simulink library "tp333079"  (Simulink 5.0)
values from neighbouring files (symbols this model uses):
  b = 1    [main_flock3.m]    (also in main_flock4.m; params_flocking_ros.m)
undefined symbols (not defined in the file or in its folder): AC, AlphaBnd, BetaBnd, CDda, CDde, CDdf, CDdr, CDM, CDmin, CGempty, CGgross, CL0, CLa, CLalphadot, Clbeta, Clda, CLde, CLdf, Cldr, CLM, CLmind, Clp, CLq, Clr, Cm0, Cma, Cmalphadot, Cmde, Cmdf, CmM, Cmq, Cnbeta, Cnda, Cndr, Cnp, Cnr, CP, CT, CYbeta, CYda, CYdr, CYp, CYr, Displacement, dmy, Engine, EulerIni, FuelFlow, FuelIni, J, Jempty, Jeng, Jgross, Jprop, MAC, MAP, MAPLim, MassIni, MaxPower, mempty ... (+26)
libraries: aerosimlib x325, simulink3 x42
(part 4 of 11)

== system tp333079/FlightGear-Compatible/Complete Aircraft ==
  CESSNA-172 : Subsystem  SimViewingDevice=off  mask(FlightGear Aircraft Model){ACName='c172', FGPath='f:\flightgear-0.8', VelocitiesIni=[60 0 0]', RatesIni=[0 0 0]', QuaternionsIni=[1 0 0 0]', PositionIni=[37.6*pi/180 -122.3*pi/180 2000]', OmegaIni=2500*pi/30, FuelIni=[50 50], GndAlt=0, tsamp=0.02}
      mask prompts: ACName "Aircraft name:"; FGPath "FlightGear path:"; VelocitiesIni "Initial velocities:"; RatesIni "Initial angular rate:"; QuaternionsIni "Initial quaternions:"; PositionIni "Initial position:"; OmegaIni "Initial engine speed:"; FuelIni "Initial fuel:"; GndAlt "Ground altitude:"; tsamp "Sample time:"
      mask help: A FlightGear aircraft model, with single piston engine, fixed-pitch propeller, and two fuel tanks.
      mask init:
      | ACen = xmlAircraft(ACName, FGPath);
      | AC = AircraftUnitConv(ACen);
      settings: Permissions=ReadWrite  RTWFcnNameOpts=Auto  RTWFileNameOpts=Auto
      mask Help:
      | A FlightGear aircraft model, with single piston engine, fixed-pitch propeller, and two fuel tanks. All parameters are in metric units. Angular measurements are in radians.
      | <P><B>Inputs:</B>
      | <LI>Control = the aircraft control vector [Flap Elevator Aileron Rudder Throttle Mixture Ignition]</LI>
      | <LI>Wind = the background wind vector, in geodetic frame [WN WE WD]</LI>
      | <LI>RST = the integrator reset flag</LI>
      | </P>
      | <P><B>Outputs:</B>
      | <LI>TAS = the true airspeed</LI>
      | <LI>AOA = the angle-of-attack</LI>
      | <LI>Position = the aircraft position [Lat Lon Alt]</LI>
      | <LI>Attitude = the aircraft attitude in Euler angles [roll pitch yaw]</LI>
      | <LI>Rates = the angular rates in body axes</LI>
      | <LI>Aero = the aerodynamic coefficients [CD CY CL Cl Cm Cn]</LI>
      | <LI>Prop = the propeller coefficients [J CT CP]</LI>
      | <LI>Engine = the engine coefficients [MAP AF FF BSFC P]</LI>
      | <LI>RPM = the engine rotation speed</LI>
      | </P>
      | <P><B>Parameters:</B>
      | <LI>Aircraft name = the name of the JSBSim aircraft</LI>
      | <LI>FlightGear path</LI>
      | <LI>Initial velocities</LI>
      | <LI>Initial angular rates</LI>
      | <LI>Initial quaternions</LI>
      | <LI>Initial position</LI>
      | <LI>Initial engine speed</LI>
      | <LI>Initial fuel mass</LI>
      | <LI>Ground altitude</LI>
      | <LI>Sample time</LI>
      | </P>
  CESSNA-182 : Subsystem  SimViewingDevice=off  mask(FlightGear Aircraft Model){ACName='c182', FGPath='f:\flightgear-0.8', VelocitiesIni=[70 0 0]', RatesIni=[0 0 0]', QuaternionsIni=[1 0 0 0]', PositionIni=[37.6*pi/180 -122.3*pi/180 500]', OmegaIni=2500*pi/30, FuelIni=[100 100], GndAlt=0, tsamp=0.02}
      mask prompts: ACName "Aircraft name:"; FGPath "FlightGear path:"; VelocitiesIni "Initial velocities:"; RatesIni "Initial angular rate:"; QuaternionsIni "Initial quaternions:"; PositionIni "Initial position:"; OmegaIni "Initial engine speed:"; FuelIni "Initial fuel:"; GndAlt "Ground altitude:"; tsamp "Sample time:"
      mask help: A FlightGear aircraft model, with single piston engine, variable-pitch propeller, and two fuel tanks.
      mask init:
      | ACen = xmlAircraft(ACName, FGPath);
      | AC = AircraftUnitConv(ACen);
      settings: Permissions=ReadWrite  RTWFcnNameOpts=Auto  RTWFileNameOpts=Auto
      mask Help:
      | A FlightGear aircraft model, with single piston engine, variable-pitch propeller, and two fuel tanks.
      | <P><B>Inputs:</B>
      | <LI>Control = the aircraft control vector [Flap Elevator Aileron Rudder Throttle Mixture Ignition Prop-pitch]</LI>
      | <LI>Wind = the background wind vector, in geodetic frame [WN WE WD]</LI>
      | <LI>RST = the integrator reset flag</LI>
      | </P>
      | <P><B>Outputs:</B>
      | <LI>TAS = the true airspeed</LI>
      | <LI>AOA = the angle-of-attack</LI>
      | <LI>Position = the aircraft position [Lat Lon Alt]</LI>
      | <LI>Attitude = the aircraft attitude in Euler angles [roll pitch yaw]</LI>
      | <LI>Rates = the angular rates in body axes</LI>
      | <LI>Aero = the aerodynamic coefficients [CD CY CL Cl Cm Cn]</LI>
      | <LI>Prop = the propeller coefficients [J CT CP]</LI>
      | <LI>Engine = the engine coefficients [MAP AF FF BSFC P]</LI>
      | <LI>RPM = the engine rotation speed</LI>
      | </P>
      | <P><B>Parameters:</B>
      | <LI>Aircraft name = the name of the JSBSim aircraft</LI>
      | <LI>FlightGear path</LI>
      | <LI>Initial velocities</LI>
      | <LI>Initial angular rates</LI>
      | <LI>Initial quaternions</LI>
      | <LI>Initial position</LI>
      | <LI>Initial engine speed</LI>
      | <LI>Initial fuel mass</LI>
      | <LI>Ground altitude</LI>
      | <LI>Sample time</LI>
      | </P>
  CESSNA-310 : Subsystem  SimViewingDevice=off  mask(FlightGear Aircraft Model){ACName='c310', FGPath='f:\flightgear-0.8', VelocitiesIni=[90 0 0]', RatesIni=[0 0 0]', QuaternionsIni=[1 0 0 0]', PositionIni=[37.6*pi/180 -122.3*pi/180 500]', OmegaIni=[2500 2500]*pi/30, FuelIni=[100 100 50 50], GndAlt=0, tsamp=0.02}
      mask prompts: ACName "Aircraft name:"; FGPath "FlightGear path:"; VelocitiesIni "Initial velocities:"; RatesIni "Initial angular rate:"; QuaternionsIni "Initial quaternions:"; PositionIni "Initial position:"; OmegaIni "Initial engine speed:"; FuelIni "Initial fuel:"; GndAlt "Ground altitude:"; tsamp "Sample time:"
      mask help: A FlightGear aircraft model, twin engine, variable-pitch propellers, and 4 fuel tanks.
      mask init:
      | ACen = xmlAircraft(ACName, FGPath);
      | AC = AircraftUnitConv(ACen);
      settings: Permissions=ReadWrite  RTWFcnNameOpts=Auto  RTWFileNameOpts=Auto
      mask Help:
      | A FlightGear aircraft model, twin engine, variable-pitch propellers, and 4 fuel tanks.
      | <P><B>Inputs:</B>
      | <LI>Control = the aircraft control vector [Flap Elevator Aileron Rudder ThrottleL MixtureL IgnitionL Prop-pitchL ThrottleR MixtureR IgnitionR Prop-pitchR]</LI>
      | <LI>Gear = the gear position flag (0 = gear up, 1 = gear down)</LI>
      | <LI>Wind = the background wind vector, in geodetic frame [WN WE WD]</LI>
      | <LI>RST = the integrator reset flag</LI>
      | </P>
      | <P><B>Outputs:</B>
      | <LI>TAS = the true airspeed</LI>
      | <LI>AOA = the angle-of-attack</LI>
      | <LI>Position = the aircraft position [Lat Lon Alt]</LI>
      | <LI>Attitude = the aircraft attitude in Euler angles [roll pitch yaw]</LI>
      | <LI>Rates = the angular rates in body axes</LI>
      | <LI>Aero = the aerodynamic coefficients [CD CY CL Cl Cm Cn]</LI>
      | <LI>PropL = the left propeller coefficients [J CT CP]</LI>
      | <LI>EngineL = the left engine coefficients [MAP AF FF BSFC P]</LI>
      | <LI>RPML = the left engine rotation speed</LI>
      | <LI>PropR = the right propeller coefficients [J CT CP]</LI>
      | <LI>EngineR = the right engine coefficients [MAP AF FF BSFC P]</LI>
      | <LI>RPMR = the right engine rotation speed</LI>
      | </P>
      | <P><B>Parameters:</B>
      | <LI>Aircraft name = the name of the JSBSim aircraft</LI>
      | <LI>FlightGear path</LI>
      | <LI>Initial velocities</LI>
      | <LI>Initial angular rates</LI>
      | <LI>Initial quaternions</LI>
      | <LI>Initial position</LI>
      | <LI>Initial engine speed [left eng, right eng]</LI>
      | <LI>Initial fuel mass [inner left, inner right, outer left, outer right]</LI>
      | <LI>Ground altitude</LI>
      | <LI>Sample time</LI>
      | </P>

== system tp333079/FlightGear-Compatible/Inertia ==
  Empty Aircraft : Subsystem  SimViewingDevice=off  mask(Empty Aircraft){Metrics=Metrics}
      mask prompts: Metrics "Aircraft metrics structure:"
      mask help: The block returns the empty aircraft inertia parameters (mass, CG location, and moments of inertia Jx Jy Jz and Jxz).
      settings: Permissions=ReadWrite  RTWFcnNameOpts=Auto  RTWFileNameOpts=Auto
      mask Help:
      | The block returns the empty aircraft inertia parameters (mass, CG location, and moments of inertia Jx Jy Jz and Jxz).
      | <P><B>Inputs:</B>
      | <LI>none</LI>
      | </P>
      | <P><B>Outputs:</B>
      | <LI>Mass = the empty aircraft mass</LI>
      | <LI>CG = the empty aircraft CG location [x y z]</LI>
      | <LI>Inertia = the empty aircraft moments of inertia [Jx Jy Jz Jxz]</LI>
      | </P>
      | <P><B>Parameters:</B>
      | <LI>Aircraft metrics structure = the Matlab structure which describes the aircraft metrics (part of the aircraft structure)</LI>
      | </P>
  Point Mass : Subsystem  SimViewingDevice=off  mask(Point Mass){PointMass=PointMass}
      mask prompts: PointMass "Point mass structure:"
      mask help: The block returns the inertia parameters of a point-mass component.
      settings: Permissions=ReadWrite  RTWFcnNameOpts=Auto  RTWFileNameOpts=Auto
      mask Help:
      | The block returns the inertia parameters of a point-mass component (mass, CG location, and moments of inertia Jx Jy Jz and Jxz).
      | <P><B>Inputs:</B>
      | <LI>none</LI>
      | </P>
      | <P><B>Outputs:</B>
      | <LI>Mass = the component mass</LI>
      | <LI>CG = the component CG location [x y z]</LI>
      | <LI>Inertia = the component moments of inertia [Jx Jy Jz Jxz]</LI>
      | </P>
      | <P><B>Parameters:</B>
      | <LI>Point mass structure = the Matlab structure which describes the point mass component (part of the aircraft structure)</LI>
      | </P>

== system tp333079/FlightGear-Compatible/Propulsion ==
  Engine : Subsystem  SimViewingDevice=off
      settings: Permissions=ReadWrite  RTWFcnNameOpts=Auto  RTWFileNameOpts=Auto
  FG Piston Engine +  Fixed-Pitch Prop : Subsystem  SimViewingDevice=off  mask(FG Piston Engine + Fixed-Pitch Prop){Eng=Engine, Thr=Thruster, pSL=pSL, TSL=TSL, OmegaIni=OmegaIni}
      mask prompts: Eng "Piston engine structure:"; Thr "Fixed-pitch prop structure:"; pSL "Sea-level pressure:"; TSL "Sea-level temperature:"; OmegaIni "Initial engine speed:"
      mask help: The block includes a piston engine, a fixed-pitch propeller and the propulsion system moment equation.
      settings: Permissions=ReadWrite  RTWFcnNameOpts=Auto  RTWFileNameOpts=Auto
      mask Help:
      | The block includes a piston engine, a fixed-pitch propeller and the propulsion system moment equation.
      | <P><B>Inputs:</B>
      | <LI>Control = the engine controls [Throttle Mixture Ignition]</LI>
      | <LI>p = the atmospheric pressure</LI>
      | <LI>T = the outside air temperature</LI>
      | <LI>rho = the air density at current altitude</LI>
      | <LI>WindAxesVel = the aircraft velocity in wind axes [airspeed sideslip angle-of-attack]</LI>
      | <LI>CGpos = the current location of the aircraft center of gravity</LI>
      | <LI>RST = the engine speed integrator reset flag</LI>
      | </P>
      | <P><B>Outputs:</B>
      | <LI>Fprop = the propulsion forces in body axes</LI>
      | <LI>Mprop = the propulsion moments with respect to the current aircraft CG</LI>
      | <LI>Omega = the engine rotation speed</LI>
      | <LI>FuelFlow = the mass fuel flow to the engine</LI>
      | <LI>EngCoeff = the engine coefficients [MAP AirFlow FuelFlow BSFC Power]</LI>
      | <LI>PropCoeff = the propeller coefficients [J CT CP]</LI>
      | </P>
      | <P><B>Parameters:</B>
      | <LI>Piston engine structure = the Matlab engine structure, which is part of the aircraft structure</LI>
      | <LI>Fixed-pitch prop structure = the Matlab thruster structure, which is part of the aircraft structure</LI>
      | <LI> Sea-level pressure and temperature</LI>
      | <LI>Initial engine speed = the initial value for the engine speed integrator</LI>
      | </P>
  FG Piston Engine +  Variable-Pitch Prop : Subsystem  SimViewingDevice=off  mask(FG Piston Engine + Variable-Pitch Prop){Eng=AC.Propulsion.Engine{1}, Thr=AC.Propulsion.Thruster{1}, pSL=101325, TSL=288.15, OmegaIni=OmegaIni}
      mask prompts: Eng "Piston engine structure:"; Thr "Fixed-pitch prop structure:"; pSL "Sea-level pressure:"; TSL "Sea-level temperature:"; OmegaIni "Initial engine speed:"
      mask help: The block includes a piston engine, a variable-pitch propeller and the propulsion system moment equation.
      settings: Permissions=ReadWrite  RTWFcnNameOpts=Auto  RTWFileNameOpts=Auto
      mask Help:
      | The block includes a piston engine, a variable-pitch propeller and the propulsion system moment equation.
      | <P><B>Inputs:</B>
      | <LI>Control = the engine controls [Throttle Mixture Ignition Prop-pitch]</LI>
      | <LI>p = the atmospheric pressure</LI>
      | <LI>T = the outside air temperature</LI>
      | <LI>rho = the air density at current altitude</LI>
      | <LI>WindAxesVel = the aircraft velocity in wind axes [airspeed sideslip angle-of-attack]</LI>
      | <LI>CGpos = the current location of the aircraft center of gravity</LI>
      | <LI>RST = the engine speed integrator reset flag</LI>
      | </P>
      | <P><B>Outputs:</B>
      | <LI>Fprop = the propulsion forces in body axes</LI>
      | <LI>Mprop = the propulsion moments with respect to the current aircraft CG</LI>
      | <LI>Omega = the engine rotation speed</LI>
      | <LI>FuelFlow = the mass fuel flow to the engine</LI>
      | <LI>EngCoeff = the engine coefficients [MAP AirFlow FuelFlow BSFC Power]</LI>
      | <LI>PropCoeff = the propeller coefficients [J CT CP]</LI>
      | </P>
      | <P><B>Parameters:</B>
      | <LI>Piston engine structure = the Matlab engine structure, which is part of the aircraft structure</LI>
      | <LI>Fixed-pitch prop structure = the Matlab thruster structure, which is part of the aircraft structure</LI>
      | <LI> Sea-level pressure and temperature</LI>
      | <LI>Initial engine speed = the initial value for the engine speed integrator</LI>
      | </P>
  Tank : Subsystem  SimViewingDevice=off
      settings: Permissions=ReadWrite  RTWFcnNameOpts=Auto  RTWFileNameOpts=Auto
  Thruster : Subsystem  SimViewingDevice=off
      settings: Permissions=ReadWrite  RTWFcnNameOpts=Auto  RTWFileNameOpts=Auto

== system tp333079/Inertia/Aircraft Inertia ==
  note: Interpolate to get current moments of inertia
  note: Interpolate to get current CG location
  note: Compute current aircraft mass
  FuelFlow : Inport  Port=1  PortDimensions=1  SampleTime=-1  DataType=auto
      settings: SignalType=auto
  RST : Inport  Port=2  PortDimensions=1  SampleTime=-1  DataType=auto
      settings: SignalType=auto
  CG Position X : Lookup  InputValues=[Mempty Mgross]  OutputValues=[CGempty(1) CGgross(1)]
  CG Position Y : Lookup  InputValues=[Mempty Mgross]  OutputValues=[CGempty(2) CGgross(2)]
  CG Position Z : Lookup  InputValues=[Mempty Mgross]  OutputValues=[CGempty(3) CGgross(3)]
  ChSign : Gain  Gain=-1  Multiplication=Element-wise(K.*u)  SaturateOnIntegerOverflow=on
  Fuel Integrator : Integrator  ExternalReset=rising  InitialConditionSource=internal  InitialCondition=FuelIni  LimitOutput=on  UpperSaturationLimit=Mgross-Mempty  LowerSaturationLimit=0  ShowSaturationPort=off  ShowStatePort=off  AbsoluteTolerance=auto
  Inertia Moment Jx : Lookup  InputValues=[Mempty Mgross]  OutputValues=[Jempty(1) Jgross(1)]
  Inertia Moment Jxz : Lookup  InputValues=[Mempty Mgross]  OutputValues=[Jempty(4) Jgross(4)]
  Inertia Moment Jy : Lookup  InputValues=[Mempty Mgross]  OutputValues=[Jempty(2) Jgross(2)]
  Inertia Moment Jz : Lookup  InputValues=[Mempty Mgross]  OutputValues=[Jempty(3) Jgross(3)]
  Mass empty : Constant  Value=Mempty
  Mux : Mux  Inputs=3
  Mux1 : Mux  Inputs=4
  Relational Operator : RelationalOperator  Operator===
  Sum : Sum  Inputs=|++  SaturateOnIntegerOverflow=on
  Fuel : Outport  Port=1
  Mass : Outport  Port=2
  CGpos : Outport  Port=3
  Inertia : Outport  Port=4
  OutofFuel : Outport  Port=5
  wires:
  Mux1/1 -> Inertia/1
  Inertia Moment Jxz/1 -> Mux1/4
  Inertia Moment Jz/1 -> Mux1/3
  Inertia Moment Jy/1 -> Mux1/2
  Inertia Moment Jx/1 -> Mux1/1
  CG Position Z/1 -> Mux/3
  CG Position Y/1 -> Mux/2
  CG Position X/1 -> Mux/1
  Sum/1 -> Mass/1, Inertia Moment Jy/1, Inertia Moment Jz/1, Inertia Moment Jxz/1, Inertia Moment Jx/1, CG Position Y/1, CG Position Z/1, CG Position X/1, Relational Operator/1
  Mass empty/1 -> Sum/2, Relational Operator/2
  Fuel Integrator/1 -> Sum/1, Fuel/1
  RST/1 -> Fuel Integrator/2
  ChSign/1 -> Fuel Integrator/1
  FuelFlow/1 -> ChSign/1
  Mux/1 -> CGpos/1
  Relational Operator/1 -> OutofFuel/1

== system tp333079/Inertia/Inertia Coefficients ==
  note: Output
  note: Get Gamma
  note: Sources
  Inertia : Inport  Port=1  PortDimensions=[4 1]  SampleTime=-1  DataType=auto
      settings: SignalType=auto
  (Jx-Jy+Jz)Jxz : Product  Inputs=2  Multiplication=Element-wise(.*)  SaturateOnIntegerOverflow=on
  (Jy-Jz)Jz : Product  Inputs=2  Multiplication=Element-wise(.*)  SaturateOnIntegerOverflow=on
  Demux : Demux  Outputs=4  BusSelectionMode=off
  Divide{,1..8} (9 alike) : Product  Inputs=*/  Multiplication=Element-wise(.*)  SaturateOnIntegerOverflow=on
  Jx(Jx-Jy) : Product  Inputs=2  Multiplication=Element-wise(.*)  SaturateOnIntegerOverflow=on
  JxJz : Product  Inputs=2  Multiplication=Element-wise(.*)  SaturateOnIntegerOverflow=on
  Jxz^2 : Math  Operator=square  OutputSignalType=auto
  Mux : Mux  Inputs=9
  One : Constant  Value=1
  Sum{,1..2,4..5} (5 alike) : Sum  Inputs=|+-  SaturateOnIntegerOverflow=on
  Sum3 : Sum  Inputs=+-+  SaturateOnIntegerOverflow=on
  Sum6 : Sum  Inputs=|++  SaturateOnIntegerOverflow=on
  Coeff : Outport  Port=1
  wires:
  Mux/1 -> Coeff/1
  Divide8/1 -> Mux/9
  Sum5/1 -> Jx(Jx-Jy)/2
  Divide7/1 -> Mux/8
  Sum6/1 -> Divide7/1
  Jx(Jx-Jy)/1 -> Sum6/1
  Divide6/1 -> Mux/7
  One/1 -> Divide6/1
  Divide5/1 -> Mux/6
  Divide4/1 -> Mux/5
  Sum4/1 -> Divide4/1
  Divide3/1 -> Mux/4
  Divide2/1 -> Mux/3
  Divide1/1 -> Mux/2
  (Jx-Jy+Jz)Jxz/1 -> Divide1/1
  Sum3/1 -> (Jx-Jy+Jz)Jxz/1
  Divide/1 -> Mux/1
  Sum2/1 -> Divide/1
  (Jy-Jz)Jz/1 -> Sum2/1
  Sum1/1 -> (Jy-Jz)Jz/1
  Sum/1 -> Divide/2, Divide1/2, Divide2/2, Divide3/2, Divide7/2, Divide8/2
  Jxz^2/1 -> Sum/2, Sum2/2, Sum6/2
  JxJz/1 -> Sum/1
  Demux/4 -> Jxz^2/1, (Jx-Jy+Jz)Jxz/2, Divide3/1, Divide5/1
  Demux/2 -> Sum1/1, Sum3/2, Divide4/2, Divide5/2, Divide6/2, Sum5/2
  Demux/1 -> JxJz/1, Sum3/1, Divide8/1, Sum4/2, Jx(Jx-Jy)/1, Sum5/1
  Inertia/1 -> Demux/1
  Demux/3 -> JxJz/2, (Jy-Jz)Jz/2, Sum1/2, Sum3/3, Divide2/1, Sum4/1

== system tp333079/Math/2pi Bound ==
  In : Inport  Port=1  PortDimensions=-1  SampleTime=-1  DataType=auto
      settings: SignalType=auto
  2pi : Constant  Value=2*pi
  Math Function : Math  Operator=mod  OutputSignalType=auto
  Out : Outport  Port=1
  wires:
  In/1 -> Math Function/1
  2pi/1 -> Math Function/2
  Math Function/1 -> Out/1

== system tp333079/Math/Cross Product ==
  Vec1 : Inport  Port=1  PortDimensions=-1  SampleTime=-1  DataType=auto
      settings: SignalType=auto
  Vec2 : Inport  Port=2  PortDimensions=-1  SampleTime=-1  DataType=auto
      settings: SignalType=auto
  Product : Product  Inputs=2  Multiplication=Element-wise(.*)  SaturateOnIntegerOverflow=on
  Product1 : Product  Inputs=2  Multiplication=Element-wise(.*)  SaturateOnIntegerOverflow=on
  Selector : Selector  InputType=Vector  ElementSrc=Internal  Elements=[2 3 1]  RowSrc=Internal  Rows=1  ColumnSrc=Internal  Columns=1  InputPortWidth=3
  Selector1 : Selector  InputType=Vector  ElementSrc=Internal  Elements=[3 1 2]  RowSrc=Internal  Rows=1  ColumnSrc=Internal  Columns=1  InputPortWidth=3
  Selector2 : Selector  InputType=Vector  ElementSrc=Internal  Elements=[3 1 2]  RowSrc=Internal  Rows=1  ColumnSrc=Internal  Columns=1  InputPortWidth=3
  Selector3 : Selector  InputType=Vector  ElementSrc=Internal  Elements=[2 3 1]  RowSrc=Internal  Rows=1  ColumnSrc=Internal  Columns=1  InputPortWidth=3
  Sum : Sum  Inputs=+-  SaturateOnIntegerOverflow=on
  ProdVec : Outport  Port=1
  wires:
  Sum/1 -> ProdVec/1
  Product1/1 -> Sum/2
  Product/1 -> Sum/1
  Selector3/1 -> Product1/2
  Selector2/1 -> Product1/1
  Selector1/1 -> Product/2
  Selector/1 -> Product/1
  Vec2/1 -> Selector3/1, Selector1/1
  Vec1/1 -> Selector2/1, Selector/1

== system tp333079/Math/Non-zero Sign ==
  In : Inport  Port=1  PortDimensions=-1  SampleTime=-1  DataType=auto
      settings: SignalType=auto
  One : Constant  Value=1
  Relational Operator : RelationalOperator  Operator===
  Sign : Signum
  Switch : Switch  Threshold=1
  Zero : Constant  Value=0
  Out : Outport  Port=1
  wires:
  Zero/1 -> Relational Operator/2
  In/1 -> Relational Operator/1, Sign/1
  Relational Operator/1 -> Switch/2
  One/1 -> Switch/1
  Sign/1 -> Switch/3
  Switch/1 -> Out/1

== system tp333079/Math/Normalization ==
  VecIn : Inport  Port=1  PortDimensions=-1  SampleTime=-1  DataType=auto
      settings: SignalType=auto
  Vector norm : Subsystem  SimViewingDevice=off
      settings: Permissions=ReadWrite  RTWFcnNameOpts=Auto  RTWFileNameOpts=Auto
      mask Type: Vector norm-2
      mask Description: Compute the 2-norm (magnitude) of a vector, |v| = sqrt(v'v)
  e/|e| : Product  Inputs=*/  Multiplication=Element-wise(.*)  SaturateOnIntegerOverflow=on
  VecOut : Outport  Port=1
  wires:
  Vector norm/1(Mag) -> e/|e|/2
  e/|e|/1 -> VecOut/1
  VecIn/1 -> Vector norm/1(Vec), e/|e|/1

== system tp333079/Math/Vector norm ==
  Vec : Inport  Port=1  PortDimensions=-1  SampleTime=-1  DataType=auto
      settings: SignalType=auto
  Dot Product : simulink3/Math/Dot Product
  Math Function : Math  Operator=sqrt  OutputSignalType=auto
  Mag : Outport  Port=1
  wires:
  Vec/1 -> Dot Product/1, Dot Product/2
  Dot Product/1 -> Math Function/1
  Math Function/1 -> Mag/1

== system tp333079/Math/Zero Offset ==
  In : Inport  Port=1  PortDimensions=-1  SampleTime=-1  DataType=auto
      settings: SignalType=auto
  Abs : Abs  SaturateOnIntegerOverflow=on
  Constant : Constant  Value=tol
  Non-zero Sign : Subsystem  SimViewingDevice=off
      settings: Permissions=ReadWrite  RTWFcnNameOpts=Auto  RTWFileNameOpts=Auto
      mask Type: Non-zero sign
      mask Description: Sign function outputs 1 for input greater than or equal to 0, and -1 otherwise.
  Product : Product  Inputs=2  Multiplication=Element-wise(.*)  SaturateOnIntegerOverflow=on
  Switch : Switch  Threshold=tol
  Out : Outport  Port=1
  wires:
  In/1 -> Switch/1, Non-zero Sign/1(In), Abs/1
  Abs/1 -> Switch/2
  Non-zero Sign/1(Out) -> Product/1
  Constant/1 -> Product/2
  Product/1 -> Switch/3
  Switch/1 -> Out/1

== system tp333079/Math/pi Bound ==
  In : Inport  Port=1  PortDimensions=-1  SampleTime=-1  DataType=auto
      settings: SignalType=auto
  2pi : Constant  Value=2*pi
  Math Function : Math  Operator=mod  OutputSignalType=auto
  Sum1 : Sum  Inputs=|+-  SaturateOnIntegerOverflow=on
  Sum2 : Sum  Inputs=|++  SaturateOnIntegerOverflow=on
  pi : Constant  Value=pi
  Out : Outport  Port=1
  wires:
  Math Function/1 -> Sum1/1
  2pi/1 -> Math Function/2
  In/1 -> Sum2/1
  Sum2/1 -> Math Function/1
  pi/1 -> Sum2/2, Sum1/2
  Sum1/1 -> Out/1

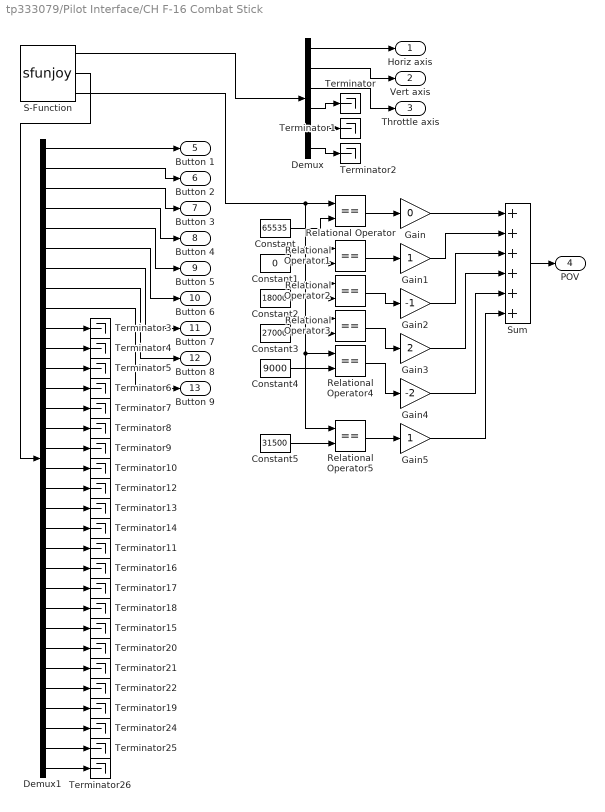
== system tp333079/Pilot Interface/CH F-16 Combat Stick ==
  Constant : Constant  Value=65535
  Constant1 : Constant  Value=0
  Constant2 : Constant  Value=18000
  Constant3 : Constant  Value=27000
  Constant4 : Constant  Value=9000
  Constant5 : Constant  Value=31500
  Demux : Demux  Outputs=6  BusSelectionMode=off
  Demux1 : Demux  Outputs=32  BusSelectionMode=off
  Gain : Gain  Gain=0  Multiplication=Element-wise(K.*u)  SaturateOnIntegerOverflow=on
  Gain1 : Gain  Gain=1  Multiplication=Element-wise(K.*u)  SaturateOnIntegerOverflow=on
  Gain2 : Gain  Gain=-1  Multiplication=Element-wise(K.*u)  SaturateOnIntegerOverflow=on
  Gain3 : Gain  Gain=2  Multiplication=Element-wise(K.*u)  SaturateOnIntegerOverflow=on
  Gain4 : Gain  Gain=-2  Multiplication=Element-wise(K.*u)  SaturateOnIntegerOverflow=on
  Gain5 : Gain  Gain=1  Multiplication=Element-wise(K.*u)  SaturateOnIntegerOverflow=on
  Relational Operator{,1..5} (6 alike) : RelationalOperator  Operator===
  S-Function : S-Function  FunctionName=sfunjoy  Parameters=tsamp  PortCounts=[]  SFunctionModules=''
  Sum : Sum  Inputs=++++++  SaturateOnIntegerOverflow=on
  Terminator{,1..22,24..26} (26 alike) : Terminator
  Horiz axis : Outport  Port=1
  Vert axis : Outport  Port=2
  Throttle axis : Outport  Port=3
  POV : Outport  Port=4
  Button 1 : Outport  Port=5
  Button 2 : Outport  Port=6
  Button 3 : Outport  Port=7
  Button 4 : Outport  Port=8
  Button 5 : Outport  Port=9
  Button 6 : Outport  Port=10
  Button 7 : Outport  Port=11
  Button 8 : Outport  Port=12
  Button 9 : Outport  Port=13
  wires:
  S-Function/1 -> Demux/1
  S-Function/2 -> Demux1/1
  S-Function/3 -> Relational Operator/1, Relational Operator1/1, Relational Operator2/1, Relational Operator3/1, Relational Operator4/1, Relational Operator5/1
  Demux/1 -> Horiz axis/1
  Demux/2 -> Vert axis/1
  Demux/3 -> Throttle axis/1
  Demux/4 -> Terminator/1
  Demux/5 -> Terminator1/1
  Demux/6 -> Terminator2/1
  Demux1/1 -> Button 1/1
  Demux1/2 -> Button 2/1
  Demux1/3 -> Button 3/1
  Demux1/4 -> Button 4/1
  Demux1/5 -> Button 5/1
  Demux1/6 -> Button 6/1
  Demux1/7 -> Button 7/1
  Demux1/8 -> Button 8/1
  Demux1/9 -> Button 9/1
  Demux1/10 -> Terminator3/1
  Demux1/11 -> Terminator4/1
  Demux1/12 -> Terminator5/1
  Demux1/13 -> Terminator6/1
  Demux1/14 -> Terminator7/1
  Demux1/15 -> Terminator8/1
  Demux1/16 -> Terminator9/1
  Demux1/17 -> Terminator10/1
  Demux1/18 -> Terminator12/1
  Demux1/19 -> Terminator13/1
  Demux1/20 -> Terminator14/1
  Demux1/21 -> Terminator11/1
  Demux1/22 -> Terminator16/1
  Demux1/23 -> Terminator17/1
  Demux1/24 -> Terminator18/1
  Demux1/25 -> Terminator15/1
  Demux1/26 -> Terminator20/1
  Demux1/27 -> Terminator21/1
  Demux1/28 -> Terminator22/1
  Demux1/29 -> Terminator19/1
  Demux1/30 -> Terminator24/1
  Demux1/31 -> Terminator25/1
  Demux1/32 -> Terminator26/1
  Constant/1 -> Relational Operator/2
  Constant1/1 -> Relational Operator1/2
  Constant2/1 -> Relational Operator2/2
  Constant3/1 -> Relational Operator3/2
  Constant4/1 -> Relational Operator4/2
  Relational Operator/1 -> Gain/1
  Relational Operator1/1 -> Gain1/1
  Relational Operator2/1 -> Gain2/1
  Relational Operator3/1 -> Gain3/1
  Relational Operator4/1 -> Gain4/1
  Relational Operator5/1 -> Gain5/1
  Constant5/1 -> Relational Operator5/2
  Gain/1 -> Sum/1
  Gain1/1 -> Sum/2
  Gain2/1 -> Sum/3
  Gain3/1 -> Sum/4
  Gain4/1 -> Sum/5
  Gain5/1 -> Sum/6
  Sum/1 -> POV/1

== system tp333079/Pilot Interface/FS Interface ==
  note: Inputs
  note: Flight Simulator Interface Function
  Position : Inport  Port=1  PortDimensions=[3 1]  SampleTime=-1  DataType=double
      settings: SignalType=auto
  Euler : Inport  Port=2  PortDimensions=[3 1]  SampleTime=-1  DataType=double
      settings: SignalType=auto
  Airspeed : Inport  Port=3  PortDimensions=1  SampleTime=-1  DataType=double
      settings: SignalType=auto
  Constant : Constant  Value=0
  Demux : Demux  Outputs=3  BusSelectionMode=off
  Mux : Mux  Inputs=3
  Mux2 : Mux  Inputs=2
  S-Function : S-Function  FunctionName=sfunflightsim  Parameters=tsamp  PortCounts=[]  SFunctionModules=''
  rad 2 deg : aerosimlib/Unit Conversion/Angular position/rad 2 deg
  rad 2 deg1 : aerosimlib/Unit Conversion/Angular position/rad 2 deg
  rad 2 deg2 : aerosimlib/Unit Conversion/Angular position/rad 2 deg
  wires:
  Mux/1 -> S-Function/1
  Mux2/1 -> S-Function/3
  Position/1 -> Demux/1
  Demux/1 -> rad 2 deg/1
  Demux/2 -> rad 2 deg1/1
  Demux/3 -> Mux/3
  rad 2 deg/1 -> Mux/1
  rad 2 deg1/1 -> Mux/2
  Euler/1 -> rad 2 deg2/1
  rad 2 deg2/1 -> S-Function/2
  Airspeed/1 -> Mux2/1
  Constant/1 -> Mux2/2

== system tp333079/Pilot Interface/FlightGear Interface ==
  note: Inputs
  note: Flight Simulator Interface Function
  Position : Inport  Port=1  PortDimensions=[3 1]  SampleTime=-1  DataType=double
      settings: SignalType=auto
  Euler : Inport  Port=2  PortDimensions=[3 1]  SampleTime=-1  DataType=double
      settings: SignalType=auto
  Airspeed : Inport  Port=3  PortDimensions=1  SampleTime=-1  DataType=double
      settings: SignalType=auto
  Constant : Constant  Value=0
  Demux : Demux  Outputs=3  BusSelectionMode=off
  Mux : Mux  Inputs=3
  Mux2 : Mux  Inputs=2
  S-Function : S-Function  FunctionName=sfunflightgear  Parameters=tsamp,hostname  PortCounts=[]  SFunctionModules=''
  wires:
  Mux/1 -> S-Function/1
  Mux2/1 -> S-Function/3
  Position/1 -> Demux/1
  Demux/1 -> Mux/1
  Demux/2 -> Mux/2
  Demux/3 -> Mux/3
  Euler/1 -> S-Function/2
  Airspeed/1 -> Mux2/1
  Constant/1 -> Mux2/2

== system tp333079/Pilot Interface/Joystick Interface ==
  S-Function : S-Function  FunctionName=sfunjoy  Parameters=tsamp  PortCounts=[]  SFunctionModules=''
  Axes : Outport  Port=1
  Buttons : Outport  Port=2
  POV : Outport  Port=3
  wires:
  S-Function/1 -> Axes/1
  S-Function/2 -> Buttons/1
  S-Function/3 -> POV/1

== system tp333079/Propulsion/Fixed-pitch Propeller ==
  note: Compute torque
  note: Interpolate propeller coefficients
  note: Compute thrust force
  note: Compute advance ratio
  note: Sources
  Airspeed : Inport  Port=1  PortDimensions=1  SampleTime=-1  DataType=double
      settings: SignalType=auto
  rho : Inport  Port=2  PortDimensions=1  SampleTime=-1  DataType=double
      settings: SignalType=auto
  Omega : Inport  Port=3  PortDimensions=1  SampleTime=-1  DataType=double
      settings: SignalType=auto
  1/pi^2 : Math  Operator=pow  OutputSignalType=auto
  1/pi^3 : Math  Operator=pow  OutputSignalType=auto
  Advance Ratio : Product  Inputs=**//  Multiplication=Element-wise(.*)  SaturateOnIntegerOverflow=on
  Coeff of Power : Lookup  InputValues=J  OutputValues=CP
  Coeff of Thrust : Lookup  InputValues=J  OutputValues=CT
  Gain : Gain  Gain=4  Multiplication=Element-wise(K.*u)  SaturateOnIntegerOverflow=on
  Gain1 : Gain  Gain=-4  Multiplication=Element-wise(K.*u)  SaturateOnIntegerOverflow=on
  Mux : Mux  Inputs=3
  Omega^2 : Math  Operator=square  OutputSignalType=auto
  Pi : Constant  Value=pi
  Prop Radius : Constant  Value=R
  R^4 : Math  Operator=pow  OutputSignalType=auto
  R^5 : Math  Operator=pow  OutputSignalType=auto
  Thrust : Product  Inputs=5  Multiplication=Element-wise(.*)  SaturateOnIntegerOverflow=on
  Torque : Product  Inputs=5  Multiplication=Element-wise(.*)  SaturateOnIntegerOverflow=on
  exp : Constant  Value=-3
  exp1 : Constant  Value=4
  exp2 : Constant  Value=5
  exp3 : Constant  Value=-2
  Fprop : Outport  Port=1
  Mprop : Outport  Port=2
  PropCoeff : Outport  Port=3
  wires:
  Mux/1 -> PropCoeff/1
  Torque/1 -> Mprop/1
  Thrust/1 -> Fprop/1
  Coeff of Thrust/1 -> Thrust/5, Mux/2
  Gain1/1 -> Torque/1
  Gain/1 -> Thrust/1
  R^5/1 -> Torque/3
  exp2/1 -> R^5/2
  R^4/1 -> Thrust/3
  exp1/1 -> R^4/2
  1/pi^3/1 -> Gain1/1
  1/pi^2/1 -> Gain/1
  exp/1 -> 1/pi^3/2
  Omega^2/1 -> Thrust/4, Torque/4
  Advance Ratio/1 -> Coeff of Thrust/1, Coeff of Power/1, Mux/1
  Prop Radius/1 -> R^5/1, R^4/1, Advance Ratio/4
  Pi/1 -> 1/pi^3/1, 1/pi^2/1, Advance Ratio/1
  Omega/1 -> Omega^2/1, Advance Ratio/3
  rho/1 -> Thrust/2, Torque/2
  Airspeed/1 -> Advance Ratio/2
  Coeff of Power/1 -> Torque/5, Mux/3
  exp3/1 -> 1/pi^2/2

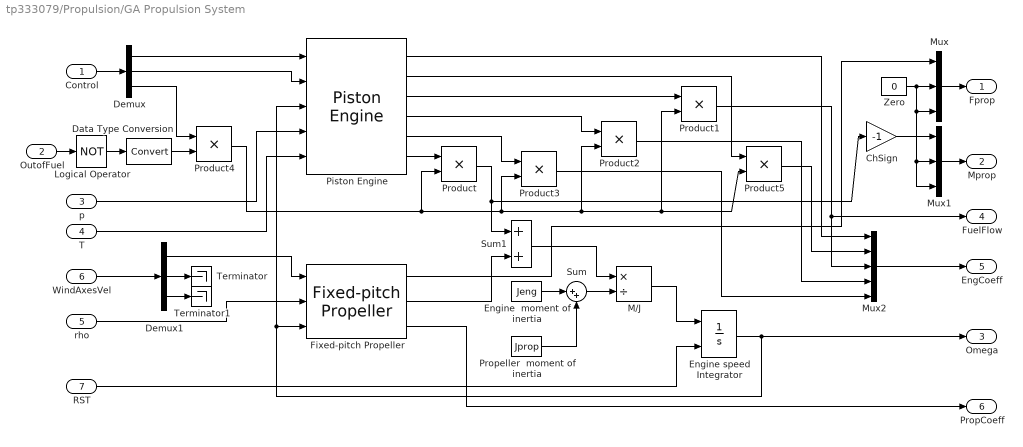
== system tp333079/Propulsion/GA Propulsion System ==
  Control : Inport  Port=1  PortDimensions=[3 1]  SampleTime=-1  DataType=auto
      settings: SignalType=auto
  OutofFuel : Inport  Port=2  PortDimensions=1  SampleTime=-1  DataType=auto
      settings: SignalType=auto
  p : Inport  Port=3  PortDimensions=1  SampleTime=-1  DataType=double
      settings: SignalType=auto
  T : Inport  Port=4  PortDimensions=1  SampleTime=-1  DataType=double
      settings: SignalType=auto
  rho : Inport  Port=5  PortDimensions=1  SampleTime=-1  DataType=double
      settings: SignalType=auto
  WindAxesVel : Inport  Port=6  PortDimensions=[3 1]  SampleTime=-1  DataType=auto
      settings: SignalType=auto
  RST : Inport  Port=7  PortDimensions=1  SampleTime=-1  DataType=double
      settings: SignalType=auto
  ChSign : Gain  Gain=-1  Multiplication=Element-wise(K.*u)  SaturateOnIntegerOverflow=on
  Data Type Conversion : DataTypeConversion  DataType=double  SaturateOnIntegerOverflow=on
  Demux : Demux  Outputs=3  BusSelectionMode=off
  Demux1 : Demux  Outputs=3  BusSelectionMode=off
  Engine  moment of inertia : Constant  Value=Jeng
  Engine speed Integrator : Integrator  ExternalReset=rising  InitialConditionSource=internal  InitialCondition=OmegaIni  LimitOutput=on  UpperSaturationLimit=inf  LowerSaturationLimit=0  ShowSaturationPort=off  ShowStatePort=off  AbsoluteTolerance=auto
  Fixed-pitch Propeller : aerosimlib/Propulsion/Fixed-pitch Propeller  J=J  CT=CT  CP=CP  R=Rprop
  Logical Operator : Logic  Operator=NOT  Inputs=2
  M/J : Product  Inputs=*/  Multiplication=Element-wise(.*)  SaturateOnIntegerOverflow=on
  Mux : Mux  Inputs=3
  Mux1 : Mux  Inputs=3
  Mux2 : Mux  Inputs=5
  Piston Engine : aerosimlib/Propulsion/Piston Engine  RPM=RPM  MAP=MAP  fflow=FuelFlow  Power=Power  TSL=TSL
  Product{,1..5} (6 alike) : Product  Inputs=2  Multiplication=Element-wise(.*)  SaturateOnIntegerOverflow=on
  Propeller  moment of inertia : Constant  Value=Jprop
  Sum : Sum  Inputs=|++  SaturateOnIntegerOverflow=on
  Sum1 : Sum  Inputs=++  SaturateOnIntegerOverflow=on
  Terminator : Terminator
  Terminator1 : Terminator
  Zero : Constant  Value=0
  Fprop : Outport  Port=1
  Mprop : Outport  Port=2
  Omega : Outport  Port=3
  FuelFlow : Outport  Port=4
  EngCoeff : Outport  Port=5
  PropCoeff : Outport  Port=6
  wires:
  T/1 -> Piston Engine/5
  p/1 -> Piston Engine/4
  Demux/2 -> Piston Engine/2
  Demux/1 -> Piston Engine/1
  Demux/3 -> Product4/1
  Logical Operator/1 -> Data Type Conversion/1
  Fixed-pitch Propeller/3 -> PropCoeff/1
  Mux2/1 -> EngCoeff/1
  Piston Engine/1 -> Mux2/1
  Product1/1 -> FuelFlow/1, Mux2/3
  Mux1/1 -> Mprop/1
  Mux/1 -> Fprop/1
  ChSign/1 -> Mux1/1
  Fixed-pitch Propeller/1 -> Mux/1
  Zero/1 -> Mux1/2, Mux1/3, Mux/3, Mux/2
  Piston Engine/3 -> Product1/1
  Piston Engine/4 -> Product2/1
  Piston Engine/5 -> Product3/1
  Piston Engine/6 -> Product/1
  Engine speed Integrator/1 -> Omega/1, Piston Engine/3, Fixed-pitch Propeller/3
  RST/1 -> Engine speed Integrator/2
  M/J/1 -> Engine speed Integrator/1
  Sum/1 -> M/J/2
  Sum1/1 -> M/J/1
  Fixed-pitch Propeller/2 -> Sum1/2
  Product/1 -> ChSign/1, Sum1/1
  Product4/1 -> Product/2, Product3/2, Product2/2, Product1/2, Product5/2
  OutofFuel/1 -> Logical Operator/1
  Propeller  moment of inertia/1 -> Sum/2
  Engine  moment of inertia/1 -> Sum/1
  rho/1 -> Fixed-pitch Propeller/2
  Demux1/1 -> Fixed-pitch Propeller/1
  Demux1/3 -> Terminator1/1
  Demux1/2 -> Terminator/1
  WindAxesVel/1 -> Demux1/1
  Control/1 -> Demux/1
  Piston Engine/2 -> Product5/1
  Product5/1 -> Mux2/2
  Product2/1 -> Mux2/4
  Product3/1 -> Mux2/5
  Data Type Conversion/1 -> Product4/2

== system tp333079/Propulsion/Piston Engine ==
  note: Compute MAP from
      | throttle area fraction
  note: Engine parameter
      | look-up tables
  note: Altitude correction for Power
  Thr : Inport  Port=1  PortDimensions=1  SampleTime=-1  DataType=double
      settings: SignalType=auto
  Mix : Inport  Port=2  PortDimensions=1  SampleTime=-1  DataType=double
      settings: SignalType=auto
  Omega : Inport  Port=3  PortDimensions=1  SampleTime=-1  DataType=double
      settings: SignalType=auto
  p : Inport  Port=4  PortDimensions=1  SampleTime=-1  DataType=double
      settings: SignalType=auto
  T : Inport  Port=5  PortDimensions=1  SampleTime=-1  DataType=double
      settings: SignalType=auto
  Engine torque : Product  Inputs=*/  Multiplication=Element-wise(.*)  SaturateOnIntegerOverflow=on
  Engine  BSFC : Product  Inputs=*/  Multiplication=Element-wise(.*)  SaturateOnIntegerOverflow=on
  Fuel flow LUT : Lookup2D  RowIndex=RPM  ColumnIndex=MAP  OutputValues=fflow
  Get air flow : Product  Inputs=2  Multiplication=Element-wise(.*)  SaturateOnIntegerOverflow=on
  Intake : Subsystem  SimViewingDevice=off  mask(Intake){MAPmin=MAP(1)}
      mask prompts: MAPmin "Minimum MAP:"
      mask help: The block computes the manifold pressure as a function of throttle area fraction, atmosphere parameters and fuel flow.
      settings: Permissions=ReadWrite  RTWFcnNameOpts=Auto  RTWFileNameOpts=Auto
  Math Function : Math  Operator=sqrt  OutputSignalType=auto
  Power LUT : Lookup2D  RowIndex=RPM  ColumnIndex=MAP  OutputValues=Power
  Power at altitude : Product  Inputs=2  Multiplication=Element-wise(.*)  SaturateOnIntegerOverflow=on
  Sea-level temperature : Constant  Value=TSL
  TSL/T : Product  Inputs=*/  Multiplication=Element-wise(.*)  SaturateOnIntegerOverflow=on
  g/hr 2 kg/s : Gain  Gain=1/1000/3600  Multiplication=Element-wise(K.*u)  SaturateOnIntegerOverflow=on
  rad/s 2 RPM : aerosimlib/Unit Conversion/Angular velocity/rad//s 2 RPM
  MAP : Outport  Port=1
  AirFlow : Outport  Port=2
  FuelFlow : Outport  Port=3
  BSFC : Outport  Port=4
  Power : Outport  Port=5
  Torque : Outport  Port=6
  wires:
  Get air flow/1 -> AirFlow/1
  Mix/1 -> Get air flow/2
  Intake/1(MAP) -> MAP/1, Power LUT/2, Fuel flow LUT/2
  g/hr 2 kg/s/1 -> Get air flow/1, FuelFlow/1
  Omega/1 -> rad/s 2 RPM/1, Engine torque/2
  rad/s 2 RPM/1 -> Fuel flow LUT/1, Power LUT/1
  Sea-level temperature/1 -> TSL/T/1
  T/1 -> TSL/T/2
  TSL/T/1 -> Math Function/1
  Power LUT/1 -> Power at altitude/1
  Math Function/1 -> Power at altitude/2
  Power at altitude/1 -> Engine torque/1, Engine  BSFC/2, Power/1
  Fuel flow LUT/1 -> Engine  BSFC/1, g/hr 2 kg/s/1
  Engine  BSFC/1 -> BSFC/1
  Engine torque/1 -> Torque/1
  Thr/1 -> Intake/1(Thr)
  p/1 -> Intake/2(p)

== system tp333079/Sensors/Analog Sensors ==
  A/D Converter : Subsystem  SimViewingDevice=off  mask(A/D Converter){Vrange=[0 5], Bits=10, tsamp=0.02}
      mask prompts: Vrange "Voltage range [min max]:"; Bits "Resolution [bits]:"; tsamp "Sample time [s]:"
      mask help: Convert the analog voltage to digital, at the specified resolution.
      mask init:
      | MinVolts = Vrange(1);
      | MaxVolts = Vrange(2);
      settings: Permissions=ReadWrite  RTWFcnNameOpts=Auto  RTWFileNameOpts=Auto
      mask Help:
      | <P>The A/D converter accepts an analog voltage as input and provides a discrete signal as an integer number (counts). The parameters that have to be set are the following:</P>
      | <LI>Voltage range = a 1x2 vector with the minimum and maximum values of the input voltage;</LI>
      | <LI>Resolution = the maximum number of counts for output, i.e. a 10-bit converter can output maximum 2^10 = 1024 counts;</LI>
      | <LI>Sample time = output count update rate.</LI>
  Analog Sensor : Subsystem  SimViewingDevice=off  mask(Analog sensor){Range=[-1 1], BiasPoint=0, BiasVolt=2.5, ScaleFactor=2.5, Bandwidth=100, NoiseSeed=[23341], NoiseCov=0.01, SampleTime=0.005}
      mask prompts: Range "Range [min max]:"; BiasPoint "Bias point:"; BiasVolt "Bias voltage:"; ScaleFactor "Scale factor:"; Bandwidth "Bandwidth at -3dB [Hz]:"; NoiseSeed "Noise seed:"; NoiseCov "Noise variance:"; SampleTime "Noise sample time:"
      mask help: Generic analog sensor featuring 2nd order dynamics, saturation limits, random walk, constant bias, and voltage conversion.
      settings: Permissions=ReadWrite  RTWFcnNameOpts=Auto  RTWFileNameOpts=Auto
      mask Help:
      | <P>This simple analog sensor block accepts the "measured" variable as input (it would normally come from the aircraft dynamic model) and it outputs an analog voltage signal which can be processed by an A/D converter block and provided to an autopilot system.</P>
      | <P><B>Block parameters:</B>
      | <LI>Range = a 1x2 vector with the minimum and maximum values that can be measured by the sensor;
      | <LI>Bias point = the zero for the measured variable (0 for most sensors);
      | <LI>Bias voltage = the voltage that the sensor will output for the bias point specified above;
      | <LI>Scale factor = the conversion factor from measured variable to voltage;
      | <LI>Bandwidth = the 2nd order dynamics bandwidth at a gain of -3dB and phase of -90 deg.;
      | <LI>Noise seed = the starting seed of the white-noise source (see Simulink help for Random Number block for more details on the seed).
      | <LI>Noise variance = the white-noise source variance.
      | <LI>Noise sample time = the sample time for the random walk white-noise source.
      | </P>

== system tp333079/Sensors/Digital Sensors ==
  GPS PV : Subsystem  SimViewingDevice=off  mask(GPS Position-Velocity){PosIni=, VelIni=, PosLag=0.1, VelLag=1.1, HPosErr=10, VPosErr=30, HVelErr=0.5, VVelErr=2, TimeConst=100, Trw=0.005}
      mask prompts: PosIni "Initial position:"; VelIni "Initial velocity:"; PosLag "Position lag [s]:"; VelLag "Velocity lag [s]:"; HPosErr "Horizontal position variance:"; VPosErr "Vertical position variance:"; HVelErr "Horizontal velocity variance:"; VVelErr "Vertical velocity variance:"; TimeConst "Noise correlation time:"; Trw "Noise sample time:"
      mask help: A simple GPS position-velocity model which includes transport delay and Gauss-Markov noise correlation.
      mask init:
      | REarth = 6371000;
      settings: Permissions=ReadWrite  RTWFcnNameOpts=Auto  RTWFileNameOpts=Auto
      mask Help:
      | <P>A simple GPS position-velocity model which includes output time-lag, Gauss-Markov noise correlation, and discrete output.</P>
      | <P><B>Inputs:</B>
      | <LI>PVIn = the 6x1 vector of aircraft position and velocity.
      | </P>
      | <P><B>Outputs:</B>
      | <LI>PVOut = the 6x1 vector of GPS position and velocity.
      | </P>
      | <P><B>Parameters:</B>
      | <LI>Initial position = the initial position output 3x1
      | <LI>Initial velocity = the initial velocity output 3x1
      | <LI>Position lag = the time lag for the position output.
      | <LI>Velocity lag = the time lag for the velocity output.
      | <LI>Horizontal position variance = the white-noise variance for the horizontal position channels (Latitude and Longitude).
      | <LI>Vertical position variance = the white-noise variance for the vertical position solution (Altitude).
      | <LI>Horizontal velocity variance = the white-noise variance for the horizontal velocity solution (VNorth, VEast).
      | <LI>Vertical velocity variance = the white noise variance for the vertical velocity solution (VDown).
      | <LI>Noise correlation time = the correlation time for the Gauss-Markov processes.
      | <LI>Noise sample time = the sample time for the white-noise sources.
      | </P>
  Single GPS Measurement : Subsystem  SimViewingDevice=off  mask(Single GPS Measurement){ValIni=, Lag=, TimeConst=, seed=, Cov=, T1=}
      mask prompts: ValIni "Initial value:"; Lag "Output lag [s]:"; TimeConst "Noise correlation time:"; seed "Noise seed:"; Cov "Noise variance:"; T1 "Noise sample time [s]:"
      mask help: GPS single channel measurement block.
      settings: Permissions=ReadWrite  RTWFcnNameOpts=Auto  RTWFileNameOpts=Auto
      mask Help:
      | <P>The block provides a single channel (position or velocity) model which includes a Gauss-Markov noise process and transport delay.</P>
      | <P><B>Parameters:</B>
      | <LI>Initial value = the initial output value.
      | <LI>Output lag = the time lag for the sensor output.
      | <LI>Noise correlation time = the time constant for the Gauss-Markov process.
      | <LI>Noise seed = the starting seed of the white-noise source.
      | <LI>Noise variance = the variance of the white-noise source output.
      | <LI>Noise sample time = the sample time of the white-noise source output.
      | <LI>Output sample time = the sample time of the block output.
      | </P>

== system tp333079/Sensors/Generic Sensors ==
  Simple Sensor (1st-order dynamics) : Subsystem  SimViewingDevice=off  mask(Simple Sensor){MaxInput=1, MinInput=-1, Lag=0.1, NoiseSeed=[23341], NoiseCov=0.01, SampleTime=0.005}
      mask prompts: MaxInput "Max value:"; MinInput "Min value:"; Lag "Output lag:"; NoiseSeed "Noise seed:"; NoiseCov "Noise variance:"; SampleTime "Noise sample time:"
      mask help: A simple sensor models which includes saturation limits, time lag and random-walk.
      settings: Permissions=ReadWrite  RTWFcnNameOpts=Auto  RTWFileNameOpts=Auto
      mask Help:
      | <P>The simple sensor with 1st-order dynamics includes time lag for the measurement, saturation limits and a random-walk correlation for the sensor noise.</P>
      | <P><B>Parameters:</B>
      | <LI>Max value = the maximum value for the input signal.
      | <LI>Min value = the minimum value for the input signal.
      | <LI>Output lag = the time lag of the sensor output.
      | <LI>Noise seed = the white-noise seed for the random walk process (refer to Simulink help for the random number block for more details on noise seed).
      | <LI>Noise variance = the variance of the white-noise source.
      | <LI>Noise sample time = the sample time of the white-noise source.
      | </P>
  Simple Sensor (2nd-order dynamics) : Subsystem  SimViewingDevice=off  mask(Simple Sensor){MaxInput=1, MinInput=-1, Bandwidth=100, NoiseSeed=[13442], NoiseCov=0.01, SampleTime=0.005}
      mask prompts: MaxInput "Max value:"; MinInput "Min value:"; Bandwidth "Bandwidth at -3dB [Hz]:"; NoiseSeed "Noise seed:"; NoiseCov "Noise variance:"; SampleTime "Noise sample time:"
      mask help: A simple sensor models which includes saturation limits, 2nd-order dynamics and random-walk.
      mask init:
      | wn = 2*pi*Bandwidth;
      | zeta = 0.5*10^(3/20);
      settings: Permissions=ReadWrite  RTWFcnNameOpts=Auto  RTWFileNameOpts=Auto
      mask Help:
      | <P>The simple sensor with 2nd-order dynamics includes limited bandwidth for the measurement, saturation limits and a random-walk correlation for the sensor noise.</P>
      | <P><B>Parameters:</B>
      | <LI>Max value = the maximum value for the input signal.
      | <LI>Min value = the minimum value for the input signal.
      | <LI>Bandwidth at -3dB = the bandwidth in Hz for a phase of -90 deg. and a gain of -3dB.
      | <LI>Noise seed = the white-noise seed for the random walk process (refer to Simulink help for the random number block for more details on noise seed).
      | <LI>Noise variance = the variance of the white-noise source.
      | <LI>Noise sample time = the sample time of the white-noise source.
      | </P>

== system tp333079/Sensors/Noise Correlation ==
  Gauss-Markov  Process : Subsystem  SimViewingDevice=off  mask(Gauss-Markov Process){beta=, seed=, Var=, T=}
      mask prompts: beta "Time constant:"; seed "White-noise seed:"; Var "Variance:"; T "Sample time:"
      mask help: The Gauss-Markov process has an exponentially decreasing autocorrelation function.
      settings: Permissions=ReadWrite  RTWFcnNameOpts=Auto  RTWFileNameOpts=Auto
      mask Help:
      | <P>The Gauss-Markov process has an exponentially decreasing autocorrelation function.</P>
      | <P><B>Block parameters:</B>
      | <LI>Time constant = the noise correlation time.
      | <LI>White-noise seed = the starting seed of the white-noise source.
      | <LI>Variance = the variance of the white-noise source.
      | <LI>Sample time = the sample time of the white-noise source.
      | </P>
  Random Walk : Subsystem  SimViewingDevice=off  mask(Random Walk){seed=, Var=, T=}
      mask prompts: seed "White-noise seed:"; Var "Variance:"; T "Sample time:"
      mask help: The random walk is also known as the Wiener process or Brownian motion. Essentially, this is the integral of a random noise signal.
      settings: Permissions=ReadWrite  RTWFcnNameOpts=Auto  RTWFileNameOpts=Auto
      mask Help:
      | <P>The random walk is also known as the Wiener process or Brownian motion. Essentially, this is the integral of a random noise signal.</P>
      | <P><B>Block parameters:</B>
      | <LI>White-noise seed = the starting seed of the white-noise source.
      | <LI>Variance = the variance of the white-noise source.
      | <LI>Sample time = the sample time of the white-noise source.
      | </P>
